simulink model "Vcu"  (R2020a)
settings: Solver=FixedStepDiscrete  StartTime=0.0  StopTime=10.0  FixedStep=ModelSimTime  RelTol=1e-3
PostLoadFcn:
  | , if any(exist('dsrtsu_mdlpostloadfcn', 'file') ~= 0), dsrtsu_mdlpostloadfcn('Execute', bdroot); end,
InitFcn:
  | , if any(exist('rtifpga_mdlclblib', 'file') ~= 0), rtifpga_mdlclblib('Init', bdroot); end,
undefined symbols (not defined in the file): rticanmm_blockfcn, rticanmm_initfcn, sigbuilder_block
libraries: rtimmsu_dsrtlib x5, commutil2 x1
(part 1 of 3)
Description:
  | Standard RTI1401 template.
  | Supported MATLAB version:  R2017b.
settings Model: Tag=RTI1401  DSRTSU_INTERNAL_RTI_VER=560  DSRTSU_INTERNAL_RTI_TYPE=rti1401  RTICANMMDATA=struct('GeneralSetupData',struct('modelroot','C:\Users\harjo\Git\MACFormulaGit\MicroAutobox\microAutoboxModels\ControlsVcu','generalsettings',struct('filesettings',struct('destfolder',struct('Name','RTICANMM_FILES','Check',1),'buildfolder',struct('Name','.','Check',1),'AbsDestfolder',struct('Name','C:\Users\harjo\Git\MACFormulaGit\MicroAutobox\microAutoboxModels\ControlsVcu\RTICANMM_FILES'),'AbsBuildfolder',struct('Name','C:\Users\harjo\Git\MACFormulaGit\MicroAutobox\microAutoboxModels\ControlsVcu'))),'options',struct('addpaths',1,'rmpaths',1,'addtrcexclusion',true,'cannavigator',struct('checkmonitoring',0),'show_usrtrc',0,'use_usrtrc',0,'addpath2usrmk',1),'advanced',struct('options',ones(1,100)),'MPSetup',{{}},'modelname','Vcu','blockdata',struct('generalsettings',struct('filesettings',struct('destfolder',struct('Name','.','Check',1),'AbsDestfolder',struct('Name','T:\TOOL_SOURCES\CANnedy\m'),'buildfolder',struct('Name','.','Check',1),'AbsBuildfolder',struct('Name','C:\MATLAB6p5\work'))),'options',struct('addpaths',1,'rmpaths',1,'addpath2usrmk',1),'modelname','rticanmmlib','modelroot','T:\TOOL_SOURCES\CANnedy\m'),'MMType','RTICANMM','block',['Vcu/RTICANMM' char(10) 'GeneralSetup'],'RTI',struct('Type','RTI1401','Ver','7.14','Date','02-May-2020'),'version','5.4.737888.359837963','userdata',struct('HostServiceChannelID',{{'Amk1','Amk2','Ams','Driver'}})))  DSRTSU_INTERNAL_RTIFPGA=160  NumberOfSteps=200  Creator=Harjot  LastModifiedBy=Harjot
settings OptimizationCC: BlockReduction=off  OptimizeBlockIOStorage=off  BufferReuse=off  GlobalBufferReuse=off  ExpressionFolding=off  LocalBlockOutputs=off  OptimizeDataStoreBuffers=off  BusAssignmentInplaceUpdate=off
settings DebuggingCC: ArithmeticOperatorsInVariantConditions=warning
settings HardwareCC: ProdBitPerPointer=32  ProdBitPerSizeT=32  ProdBitPerPtrDiffT=32  ProdLargestAtomicInteger=Integer  ProdEndianess=BigEndian  ProdWordSize=32  ProdHWDeviceType=Custom Processor->Custom  TargetIntDivRoundTo=Zero  TargetEndianess=BigEndian  TargetHWDeviceType=Custom Processor->Custom
settings SFSimCC: SimUseLocalCustomCode=off  MATLABDynamicMemAlloc=off  CustomCodeUndefinedFunction=UseInterfaceOnly
settings RTWCC: Description=dSPACE DS1401 Hardware Platform  SystemTargetFile=rti1401.tlc  MakeCommand=make_rti  TemplateMakefile=rti1401.tmf  RTWUseLocalCustomCode=off
settings CodeAppCC: MaxIdLength=128  StateflowObjectComments=on
settings STFCustomTargetCC: UtilityFuncGeneration=Shared location  ParMdlRefBuildCompliant=on  SystemTargetFile=rti1401.tlc
settings GRTTargetCC: TargetLangStandard=C89/C90 (ANSI)  UtilityFuncGeneration=Shared location  CompOptLevelCompliant=off  ConcurrentExecutionCompliant=off  CombineOutputUpdateFcns=off  MatFileLogging=off  CPPClassGenCompliant=off  UseToolchainInfoCompliant=off
settings ConfigComp: CovMetricSettings=dswe

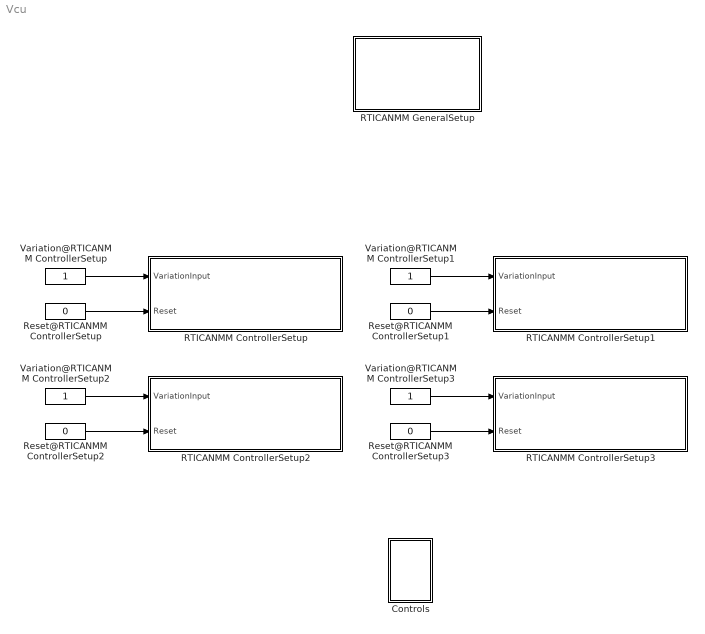
== system Vcu ==
  "Controls " : Subsystem
  RTICANMM ControllerSetup : Subsystem  InitFcn=rticanmm_blockfcn('InitFcn', 'CANnedySetup', gcb)  ClipboardFcn=rticanmm_blockfcn('ClipboardFcn', 'CANnedySetup', gcb)  mask(RTICANMM){DSProperties=struct('RTI',struct('Version',uint32(1),'BlockType',struct('isSLSource',uint8(1),'isSLSink',uint8(1),'isHWSource',uint8(0),'isHWSink',uint8(0),'isSetup',uint8(0),'isInline',uint8(1),'isNonInline',uint8(0),'isInterrupt',uint8(0),'isChannelwise',uint8(0)),'IOBoardType','RTICANMM','UnitType','RTICANMM','Identifier','BUSSETUP','DialogType','SL','BlockSet','RTICANMM','SlaveProcessor','CAN')), CANMMProperties=struct('cannedy',struct('data',struct('options',struct('controllername','Amk1','controllernameautomatic',[],'loglevel','0','checkrealtime',0,'checkchangebaudrate',0,'sampletime','1.000','CANControllerStatus',0,'NumberofStuffErr',0,'NumberofFormErr',0,'NumberofAckErr',0,'NumberofBit0Err',0,'NumberofsuccrecRX',0,'Numberofsuccsent',0,'NumberofBit1Err',0,'NumberofCRCErr',0,'NumberoflostRX',0,'Busoff',0,'Busload',0,'OperationPending',0,'TxRetryCount',3,'addtrcexclusion',true,'cannavigator',struct('checkmonitoring',0,'checkinternmonitoring',0),'show_usrtrc',0,'use_usrtrc',0,'checkchangebaudrateFD',0,'errorframegeneration',0,'efgenabled',0),'modelroot','C:\Users\harjo\Git\MACFormulaGit\MicroAutobox','generalsettings',struct('setupdata',struct('board',['CAN Type 1'],'boardno',1,'channelno',1,'Type','STD','transceiver','ISO11898-2','busconfig','0x0','feedthrough','false','resistance',struct('r120',0,'roff',1,'r16',1,'r10',0),'baudrate','500','Frequency',[24 36],'samplemode',1,'commChannelTJA1041',6,'config',struct('standard',1,'advanced',0,'register',struct('btr0','0xC0','btr1','0x6F','sp','70','sjw','3','tseg1','15','tseg2','6','brp','0','smpl','0','btr0_36','0x41','btr1_36','0x1E','sp_36','88','sjw_36','1','tseg1_36','14','tseg2_36','1','brp_36','1','smpl_36','0','btr0_64','0x43','btr1_64','0x1C','sp_64','87','sjw_64','1','tseg1_64','12','tseg2_64','1','brp_64','3','smpl_64','0')),'channelcfg',struct('INTENDISABLE','CAN_INT_DISABLE','intenable',0),'SETUPID','RTICANMM_Amk1_ID','CONTROLLER_ID','CANMM_CTL_SETUP_Amk1','mainblock_includefile','RTICANMM_SETUP_Amk1','canfdenable',0,'canfdboardselected',0,'slotno',1,'moduletype','DS4342','baudrateFD','4000','samplePoint','80','samplePointFD','80','termination','TERMINATION_OFF'),'filesettings',struct('destfolder',struct('Name','RTICANMM_FILES','Check',1),'buildfolder',struct('Name','.','Check',1))),'advanced',struct('options',ones(1,100)),'partialnetdata',struct('switchedon',0,'format','STD','idmask',['XXXXX XXXXXXXX XXXXXXXX XXXXXXXX'],'idcode','0','idfilter','0','datamaskused',0,'datalength','0','datamask','0x0000000000000000','partialnetworkenable',0)),'blk',['Vcu/RTICANMM' char(10) 'ControllerSetup'],'allgeneratedfiles',{{'C:\Users\harjo\Git\MACFormulaGit\MicroAutobox\microAutoboxModels\ControlsVcu\RTICANMM_FILES\RTICANMM_SETUP_Amk1.c','C:\Users\harjo\Git\MACFormulaGit\MicroAutobox\microAutoboxModels\ControlsVcu\RTICANMM_FILES\RTICANMM_SETUP_Amk1.h','c:\users\harjo\git\macformulagit\microautobox\microautoboxmodels\controlsvcu\rticanmm_files\rticanmm_setup_amk1.mexw64'}},'ismp',false,'BlockDataVersion','0.9.0','recreate',0,'CANnedyTag','Amk1'),'CANnedynew',0,'CANnedySettings','Amk1','GeneratedFiles',{{'C:\Users\harjo\Git\MACFormulaGit\MicroAutobox\microAutoboxModels\ControlsVcu\RTICANMM_FILES\RTICANMM_SETUP_Amk1.c','C:\Users\harjo\Git\MACFormulaGit\MicroAutobox\microAutoboxModels\ControlsVcu\RTICANMM_FILES\RTICANMM_SETUP_Amk1.h','c:\users\harjo\git\macformulagit\microautobox\microautoboxmodels\controlsvcu\rticanmm_files\rticanmm_setup_amk1.mexw64'}},'SFCN','RTICANMM_SETUP_Amk1.c','HostService',struct('Tags',struct('DATA','RTICANMM_MonitorData','TimeStampGlobal','RTICANMM_MonitoringTimeStamp','TimeStampGlobalEnable','RTICANMM_MonitoringTimeStampEnable','Enable','CANMMMonitor_Amk1','TimeStamp','MonitoringTimeStamp_Amk1'),'DATA',struct('Length',18),'Info',struct('Desc',{'ID','Service','Data1','Data2','Data3','Data4','Data5','Data6','Data7','Data8','Data9','Data10','Data11','Data12','Data13','Data14','Data15','Data16'}),'Names',struct('TimeStampGlobal','TimeStamp','TimeStampGlobalEnable','TimeStamp_Enable','Enable','Monitoring_Enable','TimeStamp','Monitoring_TimeStamp'),'ChannelID',1)), CANMMType=CANnedySetup, CANMMFolder=C:\Users\harjo\Git\MACFormulaGit\MicroAutobox\microAutoboxModels\ControlsVcu, CANMMDestFolder=RTICANMM_FILES, CANMMSettings=Amk1, CANMMSFcn=RTICANMM_SETUP_Amk1, CANMMBoard=DS1401, CANMMBoardNum=1, CANMMChannel=1}
      settings: AttributesFormatString=%<CANMMSettings>: %<CANMMBoard>_B%<CANMMBoardNum>_C%<CANMMChannel>  CopyFcn=rticanmm_blockfcn('CopyFcn', 'CANnedySetup', gcb)  DeleteFcn=rticanmm_blockfcn('DeleteFcn', 'CANnedySetup', gcb)  ModelCloseFcn=rticanmm_blockfcn('ModelCloseFcn', 'CANnedySetup', gcb)  NameChangeFcn=rticanmm_blockfcn('NameChangeFcn', 'CANnedySetup', gcb)  OpenFcn=try, rticanmm_setup_gui('create',gcb); ; catch,errordlg({lasterr, '','Please check your RTI installation.'},['Error: ' upper(bdroot)], 'replace'); end  MoveFcn=rticanmm_blockfcn('MoveFcn', 'CANnedySetup', gcb)
      mask Help: eval('rticanmm_quickstart(''create'', gcb);', 'disp(lasterr);')
      mask Display:
      | disp('RTI CAN\nMultiMessage\nControllerSetup')
      | 
      | port_label('input', 1 , 'Variation')
      | port_label('input', 2 , 'Reset')
  RTICANMM ControllerSetup1 : Subsystem  InitFcn=rticanmm_blockfcn('InitFcn', 'CANnedySetup', gcb)  ClipboardFcn=rticanmm_blockfcn('ClipboardFcn', 'CANnedySetup', gcb)  mask(RTICANMM){DSProperties=struct('RTI',struct('Version',uint32(1),'BlockType',struct('isSLSource',uint8(1),'isSLSink',uint8(1),'isHWSource',uint8(0),'isHWSink',uint8(0),'isSetup',uint8(0),'isInline',uint8(1),'isNonInline',uint8(0),'isInterrupt',uint8(0),'isChannelwise',uint8(0)),'IOBoardType','RTICANMM','UnitType','RTICANMM','Identifier','BUSSETUP','DialogType','SL','BlockSet','RTICANMM','SlaveProcessor','CAN')), CANMMProperties=struct('cannedy',struct('data',struct('options',struct('controllername','Amk2','controllernameautomatic',[],'loglevel','0','checkrealtime',0,'checkchangebaudrate',0,'sampletime','1.000','CANControllerStatus',0,'NumberofStuffErr',0,'NumberofFormErr',0,'NumberofAckErr',0,'NumberofBit0Err',0,'NumberofsuccrecRX',0,'Numberofsuccsent',0,'NumberofBit1Err',0,'NumberofCRCErr',0,'NumberoflostRX',0,'Busoff',0,'Busload',0,'OperationPending',0,'TxRetryCount',3,'addtrcexclusion',true,'cannavigator',struct('checkmonitoring',0,'checkinternmonitoring',0),'show_usrtrc',0,'use_usrtrc',0,'checkchangebaudrateFD',0,'errorframegeneration',0,'efgenabled',0),'modelroot','C:\Users\harjo\Git\MACFormulaGit\MicroAutobox','generalsettings',struct('setupdata',struct('board',['CAN Type 1'],'boardno',1,'channelno',2,'Type','STD','transceiver','ISO11898-2','busconfig','0x0','feedthrough','false','resistance',struct('r120',1,'roff',0,'r16',1,'r10',0),'baudrate','500','Frequency',[24 36],'samplemode',1,'commChannelTJA1041',6,'config',struct('standard',1,'advanced',0,'register',struct('btr0','0xC0','btr1','0x6F','sp','70','sjw','3','tseg1','15','tseg2','6','brp','0','smpl','0','btr0_36','0x41','btr1_36','0x1E','sp_36','88','sjw_36','1','tseg1_36','14','tseg2_36','1','brp_36','1','smpl_36','0','btr0_64','0x43','btr1_64','0x1C','sp_64','87','sjw_64','1','tseg1_64','12','tseg2_64','1','brp_64','3','smpl_64','0')),'channelcfg',struct('INTENDISABLE','CAN_INT_DISABLE','intenable',0),'SETUPID','RTICANMM_Amk2_ID','CONTROLLER_ID','CANMM_CTL_SETUP_Amk2','mainblock_includefile','RTICANMM_SETUP_Amk2','canfdenable',0,'canfdboardselected',0,'slotno',1,'moduletype','DS4342','baudrateFD','4000','samplePoint','80','samplePointFD','80','termination','TERMINATION_ON'),'filesettings',struct('destfolder',struct('Name','RTICANMM_FILES','Check',1),'buildfolder',struct('Name','.','Check',1))),'advanced',struct('options',ones(1,100)),'partialnetdata',struct('switchedon',0,'format','STD','idmask',['XXXXX XXXXXXXX XXXXXXXX XXXXXXXX'],'idcode','0','idfilter','0','datamaskused',0,'datalength','0','datamask','0x0000000000000000','partialnetworkenable',0)),'blk',['Vcu/RTICANMM' char(10) 'ControllerSetup1'],'allgeneratedfiles',{{'C:\Users\harjo\Git\MACFormulaGit\MicroAutobox\microAutoboxModels\ControlsVcu\RTICANMM_FILES\RTICANMM_SETUP_Amk2.c','C:\Users\harjo\Git\MACFormulaGit\MicroAutobox\microAutoboxModels\ControlsVcu\RTICANMM_FILES\RTICANMM_SETUP_Amk2.h','c:\users\harjo\git\macformulagit\microautobox\microautoboxmodels\controlsvcu\rticanmm_files\rticanmm_setup_amk2.mexw64'}},'ismp',false,'BlockDataVersion','0.9.0','recreate',0,'CANnedyTag','Amk2'),'CANnedynew',0,'CANnedySettings','Amk2','GeneratedFiles',{{'C:\Users\harjo\Git\MACFormulaGit\MicroAutobox\microAutoboxModels\ControlsVcu\RTICANMM_FILES\RTICANMM_SETUP_Amk2.c','C:\Users\harjo\Git\MACFormulaGit\MicroAutobox\microAutoboxModels\ControlsVcu\RTICANMM_FILES\RTICANMM_SETUP_Amk2.h','c:\users\harjo\git\macformulagit\microautobox\microautoboxmodels\controlsvcu\rticanmm_files\rticanmm_setup_amk2.mexw64'}},'SFCN','RTICANMM_SETUP_Amk2.c','HostService',struct('Tags',struct('DATA','RTICANMM_MonitorData','TimeStampGlobal','RTICANMM_MonitoringTimeStamp','TimeStampGlobalEnable','RTICANMM_MonitoringTimeStampEnable','Enable','CANMMMonitor_Amk2','TimeStamp','MonitoringTimeStamp_Amk2'),'DATA',struct('Length',18),'Info',struct('Desc',{'ID','Service','Data1','Data2','Data3','Data4','Data5','Data6','Data7','Data8','Data9','Data10','Data11','Data12','Data13','Data14','Data15','Data16'}),'Names',struct('TimeStampGlobal','TimeStamp','TimeStampGlobalEnable','TimeStamp_Enable','Enable','Monitoring_Enable','TimeStamp','Monitoring_TimeStamp'),'ChannelID',2)), CANMMType=CANnedySetup, CANMMFolder=C:\Users\harjo\Git\MACFormulaGit\MicroAutobox\microAutoboxModels\ControlsVcu, CANMMDestFolder=RTICANMM_FILES, CANMMSettings=Amk2, CANMMSFcn=RTICANMM_SETUP_Amk2, CANMMBoard=DS1401, CANMMBoardNum=1, CANMMChannel=2}
      settings: AttributesFormatString=%<CANMMSettings>: %<CANMMBoard>_B%<CANMMBoardNum>_C%<CANMMChannel>  CopyFcn=rticanmm_blockfcn('CopyFcn', 'CANnedySetup', gcb)  DeleteFcn=rticanmm_blockfcn('DeleteFcn', 'CANnedySetup', gcb)  ModelCloseFcn=rticanmm_blockfcn('ModelCloseFcn', 'CANnedySetup', gcb)  NameChangeFcn=rticanmm_blockfcn('NameChangeFcn', 'CANnedySetup', gcb)  OpenFcn=try, rticanmm_setup_gui('create',gcb); ; catch,errordlg({lasterr, '','Please check your RTI installation.'},['Error: ' upper(bdroot)], 'replace'); end  MoveFcn=rticanmm_blockfcn('MoveFcn', 'CANnedySetup', gcb)
      mask Help: eval('rticanmm_quickstart(''create'', gcb);', 'disp(lasterr);')
      mask Display:
      | disp('RTI CAN\nMultiMessage\nControllerSetup')
      | 
      | port_label('input', 1 , 'Variation')
      | port_label('input', 2 , 'Reset')
  RTICANMM ControllerSetup2 : Subsystem  InitFcn=rticanmm_blockfcn('InitFcn', 'CANnedySetup', gcb)  ClipboardFcn=rticanmm_blockfcn('ClipboardFcn', 'CANnedySetup', gcb)  mask(RTICANMM){DSProperties=struct('RTI',struct('Version',uint32(1),'BlockType',struct('isSLSource',uint8(1),'isSLSink',uint8(1),'isHWSource',uint8(0),'isHWSink',uint8(0),'isSetup',uint8(0),'isInline',uint8(1),'isNonInline',uint8(0),'isInterrupt',uint8(0),'isChannelwise',uint8(0)),'IOBoardType','RTICANMM','UnitType','RTICANMM','Identifier','BUSSETUP','DialogType','SL','BlockSet','RTICANMM','SlaveProcessor','CAN')), CANMMProperties=struct('cannedy',struct('data',struct('options',struct('controllername','Ams','controllernameautomatic',[],'loglevel','0','checkrealtime',0,'checkchangebaudrate',0,'sampletime','1.000','CANControllerStatus',0,'NumberofStuffErr',0,'NumberofFormErr',0,'NumberofAckErr',0,'NumberofBit0Err',0,'NumberofsuccrecRX',0,'Numberofsuccsent',0,'NumberofBit1Err',0,'NumberofCRCErr',0,'NumberoflostRX',0,'Busoff',0,'Busload',0,'OperationPending',0,'TxRetryCount',3,'addtrcexclusion',true,'cannavigator',struct('checkmonitoring',0,'checkinternmonitoring',0),'show_usrtrc',0,'use_usrtrc',0,'checkchangebaudrateFD',0,'errorframegeneration',0,'efgenabled',0),'modelroot','C:\Users\harjo\Git\MACFormulaGit\MicroAutobox','generalsettings',struct('setupdata',struct('board',['CAN Type 1'],'boardno',2,'channelno',1,'Type','STD','transceiver','ISO11898-2','busconfig','0x0','feedthrough','false','resistance',struct('r120',0,'roff',1,'r16',1,'r10',0),'baudrate','500','Frequency',[24 36],'samplemode',1,'commChannelTJA1041',6,'config',struct('standard',1,'advanced',0,'register',struct('btr0','0xC0','btr1','0x6F','sp','70','sjw','3','tseg1','15','tseg2','6','brp','0','smpl','0','btr0_36','0x41','btr1_36','0x1E','sp_36','88','sjw_36','1','tseg1_36','14','tseg2_36','1','brp_36','1','smpl_36','0','btr0_64','0x43','btr1_64','0x1C','sp_64','87','sjw_64','1','tseg1_64','12','tseg2_64','1','brp_64','3','smpl_64','0')),'channelcfg',struct('INTENDISABLE','CAN_INT_DISABLE','intenable',0),'SETUPID','RTICANMM_Ams_ID','CONTROLLER_ID','CANMM_CTL_SETUP_Ams','mainblock_includefile','RTICANMM_SETUP_Ams','canfdenable',0,'canfdboardselected',0,'slotno',1,'moduletype','DS4342','baudrateFD','4000','samplePoint','80','samplePointFD','80','termination','TERMINATION_OFF'),'filesettings',struct('destfolder',struct('Name','RTICANMM_FILES','Check',1),'buildfolder',struct('Name','.','Check',1))),'advanced',struct('options',ones(1,100)),'partialnetdata',struct('switchedon',0,'format','STD','idmask',['XXXXX XXXXXXXX XXXXXXXX XXXXXXXX'],'idcode','0','idfilter','0','datamaskused',0,'datalength','0','datamask','0x0000000000000000','partialnetworkenable',0)),'blk',['Vcu/RTICANMM' char(10) 'ControllerSetup2'],'allgeneratedfiles',{{'C:\Users\harjo\Git\MACFormulaGit\MicroAutobox\microAutoboxModels\ControlsVcu\RTICANMM_FILES\RTICANMM_SETUP_Ams.c','C:\Users\harjo\Git\MACFormulaGit\MicroAutobox\microAutoboxModels\ControlsVcu\RTICANMM_FILES\RTICANMM_SETUP_Ams.h','c:\users\harjo\git\macformulagit\microautobox\microautoboxmodels\controlsvcu\rticanmm_files\rticanmm_setup_ams.mexw64'}},'ismp',false,'BlockDataVersion','0.9.0','recreate',0,'CANnedyTag','Ams'),'CANnedynew',0,'CANnedySettings','Ams','GeneratedFiles',{{'C:\Users\harjo\Git\MACFormulaGit\MicroAutobox\microAutoboxModels\ControlsVcu\RTICANMM_FILES\RTICANMM_SETUP_Ams.c','C:\Users\harjo\Git\MACFormulaGit\MicroAutobox\microAutoboxModels\ControlsVcu\RTICANMM_FILES\RTICANMM_SETUP_Ams.h','c:\users\harjo\git\macformulagit\microautobox\microautoboxmodels\controlsvcu\rticanmm_files\rticanmm_setup_ams.mexw64'}},'SFCN','RTICANMM_SETUP_Ams.c','HostService',struct('Tags',struct('DATA','RTICANMM_MonitorData','TimeStampGlobal','RTICANMM_MonitoringTimeStamp','TimeStampGlobalEnable','RTICANMM_MonitoringTimeStampEnable','Enable','CANMMMonitor_Ams','TimeStamp','MonitoringTimeStamp_Ams'),'DATA',struct('Length',18),'Info',struct('Desc',{'ID','Service','Data1','Data2','Data3','Data4','Data5','Data6','Data7','Data8','Data9','Data10','Data11','Data12','Data13','Data14','Data15','Data16'}),'Names',struct('TimeStampGlobal','TimeStamp','TimeStampGlobalEnable','TimeStamp_Enable','Enable','Monitoring_Enable','TimeStamp','Monitoring_TimeStamp'),'ChannelID',3)), CANMMType=CANnedySetup, CANMMFolder=C:\Users\harjo\Git\MACFormulaGit\MicroAutobox\microAutoboxModels\ControlsVcu, CANMMDestFolder=RTICANMM_FILES, CANMMSettings=Ams, CANMMSFcn=RTICANMM_SETUP_Ams, CANMMBoard=DS1401, CANMMBoardNum=2, CANMMChannel=1}
      settings: AttributesFormatString=%<CANMMSettings>: %<CANMMBoard>_B%<CANMMBoardNum>_C%<CANMMChannel>  CopyFcn=rticanmm_blockfcn('CopyFcn', 'CANnedySetup', gcb)  DeleteFcn=rticanmm_blockfcn('DeleteFcn', 'CANnedySetup', gcb)  ModelCloseFcn=rticanmm_blockfcn('ModelCloseFcn', 'CANnedySetup', gcb)  NameChangeFcn=rticanmm_blockfcn('NameChangeFcn', 'CANnedySetup', gcb)  OpenFcn=try, rticanmm_setup_gui('create',gcb); ; catch,errordlg({lasterr, '','Please check your RTI installation.'},['Error: ' upper(bdroot)], 'replace'); end  MoveFcn=rticanmm_blockfcn('MoveFcn', 'CANnedySetup', gcb)
      mask Help: eval('rticanmm_quickstart(''create'', gcb);', 'disp(lasterr);')
      mask Display:
      | disp('RTI CAN\nMultiMessage\nControllerSetup')
      | 
      | port_label('input', 1 , 'Variation')
      | port_label('input', 2 , 'Reset')
  RTICANMM ControllerSetup3 : Subsystem  InitFcn=rticanmm_blockfcn('InitFcn', 'CANnedySetup', gcb)  ClipboardFcn=rticanmm_blockfcn('ClipboardFcn', 'CANnedySetup', gcb)  mask(RTICANMM){DSProperties=struct('RTI',struct('Version',uint32(1),'BlockType',struct('isSLSource',uint8(1),'isSLSink',uint8(1),'isHWSource',uint8(0),'isHWSink',uint8(0),'isSetup',uint8(0),'isInline',uint8(1),'isNonInline',uint8(0),'isInterrupt',uint8(0),'isChannelwise',uint8(0)),'IOBoardType','RTICANMM','UnitType','RTICANMM','Identifier','BUSSETUP','DialogType','SL','BlockSet','RTICANMM','SlaveProcessor','CAN')), CANMMProperties=struct('cannedy',struct('data',struct('options',struct('controllername','Driver','controllernameautomatic',[],'loglevel','0','checkrealtime',0,'checkchangebaudrate',0,'sampletime','1.000','CANControllerStatus',0,'NumberofStuffErr',0,'NumberofFormErr',0,'NumberofAckErr',0,'NumberofBit0Err',0,'NumberofsuccrecRX',0,'Numberofsuccsent',0,'NumberofBit1Err',0,'NumberofCRCErr',0,'NumberoflostRX',0,'Busoff',0,'Busload',0,'OperationPending',0,'TxRetryCount',3,'addtrcexclusion',true,'cannavigator',struct('checkmonitoring',0,'checkinternmonitoring',0),'show_usrtrc',0,'use_usrtrc',0,'checkchangebaudrateFD',0,'errorframegeneration',0,'efgenabled',0),'modelroot','C:\Users\harjo\Git\MACFormulaGit\MicroAutobox','generalsettings',struct('setupdata',struct('board',['CAN Type 1'],'boardno',2,'channelno',2,'Type','STD','transceiver','ISO11898-2','busconfig','0x0','feedthrough','false','resistance',struct('r120',1,'roff',0,'r16',1,'r10',0),'baudrate','500','Frequency',[24 36],'samplemode',1,'commChannelTJA1041',6,'config',struct('standard',1,'advanced',0,'register',struct('btr0','0xC0','btr1','0x6F','sp','70','sjw','3','tseg1','15','tseg2','6','brp','0','smpl','0','btr0_36','0x41','btr1_36','0x1E','sp_36','88','sjw_36','1','tseg1_36','14','tseg2_36','1','brp_36','1','smpl_36','0','btr0_64','0x43','btr1_64','0x1C','sp_64','87','sjw_64','1','tseg1_64','12','tseg2_64','1','brp_64','3','smpl_64','0')),'channelcfg',struct('INTENDISABLE','CAN_INT_DISABLE','intenable',0),'SETUPID','RTICANMM_Driver_ID','CONTROLLER_ID','CANMM_CTL_SETUP_Driver','mainblock_includefile','RTICANMM_SETUP_Driver','canfdenable',0,'canfdboardselected',0,'slotno',1,'moduletype','DS4342','baudrateFD','4000','samplePoint','80','samplePointFD','80','termination','TERMINATION_ON'),'filesettings',struct('destfolder',struct('Name','RTICANMM_FILES','Check',1),'buildfolder',struct('Name','.','Check',1))),'advanced',struct('options',ones(1,100)),'partialnetdata',struct('switchedon',0,'format','STD','idmask',['XXXXX XXXXXXXX XXXXXXXX XXXXXXXX'],'idcode','0','idfilter','0','datamaskused',0,'datalength','0','datamask','0x0000000000000000','partialnetworkenable',0)),'blk',['Vcu/RTICANMM' char(10) 'ControllerSetup3'],'allgeneratedfiles',{{'C:\Users\harjo\Git\MACFormulaGit\MicroAutobox\microAutoboxModels\ControlsVcu\RTICANMM_FILES\RTICANMM_SETUP_Driver.c','C:\Users\harjo\Git\MACFormulaGit\MicroAutobox\microAutoboxModels\ControlsVcu\RTICANMM_FILES\RTICANMM_SETUP_Driver.h','c:\users\harjo\git\macformulagit\microautobox\microautoboxmodels\controlsvcu\rticanmm_files\rticanmm_setup_driver.mexw64'}},'ismp',false,'BlockDataVersion','0.9.0','recreate',0,'CANnedyTag','Driver'),'CANnedynew',0,'CANnedySettings','Driver','GeneratedFiles',{{'C:\Users\harjo\Git\MACFormulaGit\MicroAutobox\microAutoboxModels\ControlsVcu\RTICANMM_FILES\RTICANMM_SETUP_Driver.c','C:\Users\harjo\Git\MACFormulaGit\MicroAutobox\microAutoboxModels\ControlsVcu\RTICANMM_FILES\RTICANMM_SETUP_Driver.h','c:\users\harjo\git\macformulagit\microautobox\microautoboxmodels\controlsvcu\rticanmm_files\rticanmm_setup_driver.mexw64'}},'SFCN','RTICANMM_SETUP_Driver.c','HostService',struct('Tags',struct('DATA','RTICANMM_MonitorData','TimeStampGlobal','RTICANMM_MonitoringTimeStamp','TimeStampGlobalEnable','RTICANMM_MonitoringTimeStampEnable','Enable','CANMMMonitor_Driver','TimeStamp','MonitoringTimeStamp_Driver'),'DATA',struct('Length',18),'Info',struct('Desc',{'ID','Service','Data1','Data2','Data3','Data4','Data5','Data6','Data7','Data8','Data9','Data10','Data11','Data12','Data13','Data14','Data15','Data16'}),'Names',struct('TimeStampGlobal','TimeStamp','TimeStampGlobalEnable','TimeStamp_Enable','Enable','Monitoring_Enable','TimeStamp','Monitoring_TimeStamp'),'ChannelID',4)), CANMMType=CANnedySetup, CANMMFolder=C:\Users\harjo\Git\MACFormulaGit\MicroAutobox\microAutoboxModels\ControlsVcu, CANMMDestFolder=RTICANMM_FILES, CANMMSettings=Driver, CANMMSFcn=RTICANMM_SETUP_Driver, CANMMBoard=DS1401, CANMMBoardNum=2, CANMMChannel=2}
      settings: AttributesFormatString=%<CANMMSettings>: %<CANMMBoard>_B%<CANMMBoardNum>_C%<CANMMChannel>  CopyFcn=rticanmm_blockfcn('CopyFcn', 'CANnedySetup', gcb)  DeleteFcn=rticanmm_blockfcn('DeleteFcn', 'CANnedySetup', gcb)  ModelCloseFcn=rticanmm_blockfcn('ModelCloseFcn', 'CANnedySetup', gcb)  NameChangeFcn=rticanmm_blockfcn('NameChangeFcn', 'CANnedySetup', gcb)  OpenFcn=try, rticanmm_setup_gui('create',gcb); ; catch,errordlg({lasterr, '','Please check your RTI installation.'},['Error: ' upper(bdroot)], 'replace'); end  MoveFcn=rticanmm_blockfcn('MoveFcn', 'CANnedySetup', gcb)
      mask Help: eval('rticanmm_quickstart(''create'', gcb);', 'disp(lasterr);')
      mask Display:
      | disp('RTI CAN\nMultiMessage\nControllerSetup')
      | 
      | port_label('input', 1 , 'Variation')
      | port_label('input', 2 , 'Reset')
  RTICANMM GeneralSetup : Subsystem  InitFcn=rticanmm_initfcn(gcb, 'CANnedySettings')  ClipboardFcn=rticanmm_blockfcn('ClipboardFcn', 'CANnedySettings', gcb)  mask(RTICANMM){DSProperties=struct('RTI',struct('Version',uint32(1),'BlockType',struct('isSLSource',uint8(1),'isSLSink',uint8(1),'isHWSource',uint8(0),'isHWSink',uint8(0),'isSetup',uint8(0),'isInline',uint8(1),'isNonInline',uint8(0),'isInterrupt',uint8(0),'isChannelwise',uint8(0)),'IOBoardType','RTICANMM','UnitType','RTICANMM','Identifier','GENERALSETUP','DialogType','SL','BlockSet','RTICANMM','SlaveProcessor','CAN')), CANMMDestFolder=RTICANMM_FILES, CANMMBuildDir=., CANMMAddPaths=on, CANMMAddpathUserMake=on, CANMMRemovePathOnclose=on, CANMMType=CANnedySettings, CANMMProperties=struct('modelroot','C:\Users\harjo\Git\MACFormulaGit\MicroAutobox\microAutoboxModels\ControlsVcu','generalsettings',struct('filesettings',struct('destfolder',struct('Name','RTICANMM_FILES','Check',1),'buildfolder',struct('Name','.','Check',1),'AbsDestfolder',struct('Name','C:\Users\harjo\Git\MACFormulaGit\MicroAutobox\microAutoboxModels\ControlsVcu\RTICANMM_FILES'),'AbsBuildfolder',struct('Name','C:\Users\harjo\Git\MACFormulaGit\MicroAutobox\microAutoboxModels\ControlsVcu'))),'options',struct('addpaths',1,'rmpaths',1,'addtrcexclusion',true,'cannavigator',struct('checkmonitoring',0),'show_usrtrc',0,'use_usrtrc',0,'addpath2usrmk',1),'advanced',struct('options',ones(1,100)),'MPSetup',{{}},'modelname','Vcu','blockdata',struct('generalsettings',struct('filesettings',struct('destfolder',struct('Name','.','Check',1),'AbsDestfolder',struct('Name','T:\TOOL_SOURCES\CANnedy\m'),'buildfolder',struct('Name','.','Check',1),'AbsBuildfolder',struct('Name','C:\MATLAB6p5\work'))),'options',struct('addpaths',1,'rmpaths',1,'addpath2usrmk',1),'modelname','rticanmmlib','modelroot','T:\TOOL_SOURCES\CANnedy\m'),'MMType','RTICANMM','block',['Vcu/RTICANMM' char(10) 'GeneralSetup'],'RTI',struct('Type','RTI1401','Ver','7.14','Date','02-May-2020'),'version','5.4.737888.359837963','userdata',struct('HostServiceChannelID',{{'Amk1','Amk2','Ams','Driver'}}))}
      mask prompts: CANMMDestFolder "Destination Folder for generated Files:"; CANMMBuildDir "Build Directory (*_usr.mk, *_usr.trc)"; CANMMAddPaths "Add Paths automatically"; CANMMAddpathUserMake "Add Paths to UserMake-File"; CANMMRemovePathOnclose "Remove added Path on ModelClose"
      mask init:
      | rticanmm_initfcn(gcb,'CANnedyGeneralSettings')
      settings: CopyFcn=rticanmm_blockfcn('CopyFcn', 'CANnedySettings', gcb)  DeleteFcn=rticanmm_blockfcn('DeleteFcn', 'CANnedySettings', gcb)  ModelCloseFcn=rticanmm_blockfcn('CloseFcn', 'CANnedyGeneralSettings', gcb)  NameChangeFcn=rticanmm_blockfcn('NameChangeFcn', 'CANnedySettings', gcb)  OpenFcn=try, rticanmm_gs_gui('create',gcb), ; catch,errordlg({lasterr, '','Please check your RTI installation.'},['Error: ' upper(bdroot)], 'replace'); end  MoveFcn=rticanmm_blockfcn('MoveFcn', 'CANnedySettings', gcb)
      mask Help: eval('rticanmm_quickstart(''create'', gcb);', 'disp(lasterr);')
      mask Display: disp(sprintf(['RTI CAN\nMultiMessage\nGeneralSetup']))
  Reset@RTICANMM ControllerSetup{,1..3} (4 alike) : Constant  Value=0  OutDataTypeStr=boolean
  Variation@RTICANMM ControllerSetup{,1..3} (4 alike) : Constant  OutDataTypeStr=uint8
  wires:
  Variation@RTICANMM ControllerSetup/1 -> RTICANMM ControllerSetup/1(VariationInput)
  Reset@RTICANMM ControllerSetup/1 -> RTICANMM ControllerSetup/2(Reset)
  Variation@RTICANMM ControllerSetup1/1 -> RTICANMM ControllerSetup1/1(VariationInput)
  Reset@RTICANMM ControllerSetup1/1 -> RTICANMM ControllerSetup1/2(Reset)
  Variation@RTICANMM ControllerSetup2/1 -> RTICANMM ControllerSetup2/1(VariationInput)
  Reset@RTICANMM ControllerSetup2/1 -> RTICANMM ControllerSetup2/2(Reset)
  Variation@RTICANMM ControllerSetup3/1 -> RTICANMM ControllerSetup3/1(VariationInput)
  Reset@RTICANMM ControllerSetup3/1 -> RTICANMM ControllerSetup3/2(Reset)
